simulink library "Ampere_Library"  (R2022b)
settings: Solver=FixedStepDiscrete  StartTime=0  StopTime=10.0  RelTol=1e-3  EnableMultiTasking=on
undefined symbols (not defined in the file or in its folder): A_INST_double, Dem_EventStatusType, ECU_AMBIENT_TEMPERATURE, SET_ECU_AMBIENT_TEMPERATURE, SlDemoSign, Std_ReturnType
libraries: simulink x13
(part 7 of 10)

== system Ampere_Library/User_Defined_Libraries/Discrete/A_1stOrder_Derivative_Filter ==
  note: A_DivisionByZero
  note: A_UnitDelayExternalIC
  note: Refer Mask Description of this Library block for detailed information.
  In : Inport
  Init_val : Inport  Port=2
  Tau : Inport  Port=3
  Te : Inport  Port=4
  Reset : Inport  Port=5
  Abs1 : Abs  RndMeth=Zero  SaturateOnIntegerOverflow=off
  ConstZero : Constant  Value=ConstZero  OutDataTypeStr=Inherit: Inherit via back propagation
  ConstZero1 : Constant  Value=ConstZero  OutDataTypeStr=Inherit: Inherit via back propagation
  Divide : Product  Inputs=*/  OutDataTypeStr=Inherit: Inherit via back propagation  RndMeth=Zero
  FixPtUnitDelay2 : UnitDelay  DisableCoverage=on  InitialCondition=false  SampleTime=-1  HasFrameUpgradeWarning=on
      settings: AttributesFormatString=Init = %<InitialCondition>
  FixPt_Unit_Delay1 : UnitDelay  DisableCoverage=on  InitialCondition=UDEIC_zero  SampleTime=-1  HasFrameUpgradeWarning=on
      settings: AttributesFormatString=Init = %<InitialCondition>
  Init : Switch  Criteria=u2 ~= 0  RndMeth=Zero  ZeroCross=off  SaturateOnIntegerOverflow=off
  LogicalOperator : Logic  Operator=OR  OutDataTypeStr=boolean
  MinMax1 : MinMax  Function=max  Inputs=2  InputSameDT=on  RndMeth=Zero
  Product : Product  InputSameDT=on  OutDataTypeStr=Inherit: Inherit via back propagation  RndMeth=Zero
  RelationalOperator : RelationalOperator  Operator=>  OutDataTypeStr=boolean  RndMeth=Zero
  Sum : Sum  InputSameDT=on  RndMeth=Zero
  Sum1 : Sum  Inputs=+-  InputSameDT=on  RndMeth=Zero
  Sum2 : Sum  InputSameDT=on  OutDataTypeStr=Inherit: Inherit via back propagation  RndMeth=Zero
  Switch : Switch  Criteria=u2 ~= 0  RndMeth=Zero  SaturateOnIntegerOverflow=off
  Switch2 : Switch  Criteria=u2 ~= 0  RndMeth=Zero  SaturateOnIntegerOverflow=off
  Switch3 : Switch  Criteria=u2 ~= 0  RndMeth=Zero  SaturateOnIntegerOverflow=off
  UnitDelay1 : UnitDelay  InitialCondition=true  SampleTime=-1  HasFrameUpgradeWarning=on
      settings: AttributesFormatString=Init = %<InitialCondition>
  false : Constant  Value=false
  tol : Constant  Value=tol  OutDataTypeStr=Inherit: Inherit via back propagation
  true : Constant  DisableCoverage=on  Value=true
  Out : Outport
  dOut_by_dt : Outport  Port=2
  wires:
  ConstZero1/1 -> Switch3/1
  Product/1 -> Sum2/1
  Init/1 -> Sum1/2, Sum2/2
  false/1 -> UnitDelay1/1
  UnitDelay1/1 -> LogicalOperator/1
  Sum2/1 -> Switch2/3
  Tau/1 -> Sum/1
  Sum/1 -> MinMax1/1
  Reset/1 -> LogicalOperator/2
  In/1 -> Sum1/1
  Switch3/1 -> dOut_by_dt/1
  Switch/1 -> Switch3/3, Product/1
  LogicalOperator/1 -> Switch2/2, Switch3/2
  Init_val/1 -> Init/3, [Init_val]
  FixPt_Unit_Delay1/1 -> Init/1
  FixPtUnitDelay2/1 -> Init/2
  true/1 -> FixPtUnitDelay2/1
  Switch2/1 -> FixPt_Unit_Delay1/1, Out/1
  Abs1/1 -> RelationalOperator/1
  MinMax1/1 -> Divide/2, Abs1/1
  ConstZero/1 -> Switch/3
  tol/1 -> RelationalOperator/2
  Divide/1 -> Switch/1
  RelationalOperator/1 -> Switch/2
  Sum1/1 -> Divide/1
  [Init_val] -> Switch2/1
  Te/1 -> Product/2, MinMax1/2, Sum/2

== system Ampere_Library/User_Defined_Libraries/Discrete/A_DiagnosticFilter ==
  note: Refer Mask Description of this Library block for detailed information.
  Reset : Inport  OutDataTypeStr=boolean
      settings: AttributesFormatString=DT = %<OutDataTypeStr>
  in : Inport  Port=2
  Diagnostic_Filter : Subsystem  TreatAsAtomicUnit=on
      settings: RTWSystemCode=Inline
  out : Outport
  DiagnosticStatus : Outport  Port=2
  wires:
  Reset/1 -> Diagnostic_Filter/Enable
  Diagnostic_Filter/2(DiagnosticStatus) -> DiagnosticStatus/1
  Diagnostic_Filter/1(out) -> out/1
  in/1 -> Diagnostic_Filter/1(in)

== system Ampere_Library/User_Defined_Libraries/Discrete/A_DiscreteInt_Ext_SAT ==
  note: Detect Increase
  note: Refer Mask Description of this Library block for detailed information.
  in : Inport
  reset : Inport  Port=2
  ic : Inport  Port=3
  Ts : Inport  Port=4
  sat_max : Inport  Port=5
  sat_min : Inport  Port=6
  Logical_Operator : Logic  OutDataTypeStr=boolean
  Logical_Operator1 : Logic  Operator=NOT  OutDataTypeStr=boolean
  MinMax : MinMax  Function=max  Inputs=2  InputSameDT=on  RndMeth=Zero
      settings: AttributesFormatString=SAT = %<SaturateOnIntegerOverflow>\n
  MinMax1 : MinMax  Inputs=2  InputSameDT=on  RndMeth=Zero
      settings: AttributesFormatString=SAT = %<SaturateOnIntegerOverflow>\n
  Product : Product  InputSameDT=on  OutDataTypeStr=Inherit: Inherit via back propagation  RndMeth=Zero
      settings: AttributesFormatString=SAT = %<SaturateOnIntegerOverflow>\n
  Sum1 : Sum  InputSameDT=on  RndMeth=Zero
      settings: AttributesFormatString=SAT = %<SaturateOnIntegerOverflow>
  Switch : Switch  Criteria=u2 ~= 0  RndMeth=Zero  SaturateOnIntegerOverflow=off
      settings: AttributesFormatString=SAT = %<SaturateOnIntegerOverflow>
  Unit_Delay : UnitDelay  InitialCondition=Input_IC  SampleTime=-1  HasFrameUpgradeWarning=on
      settings: AttributesFormatString=Init = %<InitialCondition>
  Unit_Delay1 : UnitDelay  InitialCondition=IniVal  SampleTime=-1  HasFrameUpgradeWarning=on
      settings: AttributesFormatString=Init = %<InitialCondition>\n
  Unit_Delay2 : UnitDelay  InitialCondition=false  SampleTime=-1  HasFrameUpgradeWarning=on
      settings: AttributesFormatString=Init = %<InitialCondition>\n
  out : Outport
  wires:
  sat_max/1 -> MinMax1/1
  Unit_Delay1/1 -> Sum1/2
  Product/1 -> Sum1/1
  Unit_Delay/1 -> Product/1
  Ts/1 -> Product/2
  in/1 -> Unit_Delay/1
  Logical_Operator1/1 -> Logical_Operator/2
  Unit_Delay2/1 -> Logical_Operator1/1
  reset/1 -> Logical_Operator/1, Unit_Delay2/1
  ic/1 -> Switch/1
  Sum1/1 -> Switch/3
  MinMax/1 -> MinMax1/2
  MinMax1/1 -> Unit_Delay1/1, out/1
  Switch/1 -> MinMax/2
  Logical_Operator/1 -> Switch/2
  sat_min/1 -> MinMax/1

== system Ampere_Library/User_Defined_Libraries/Discrete/A_DiscreteIntegrator ==
  note: Unused data depending
      | of mask configuration
  note: Refer Mask Description of this Library block for detailed information.
  note: tmp = in[k-1] * K * Ts
  note: y[k] = tmp + y[k-1]
  note: y[k]
  note: GotoTag updated through mask callback
  in : Inport
  reset : Inport  Port=2
  ic : Inport  Port=3
  DataTypeDuplicate : DataTypeDuplicate  NumInputPorts=4
  K : Constant  Value=K  OutDataTypeStr=Inherit: Inherit via back propagation
  Logical_Operator : Logic  OutDataTypeStr=boolean
  Logical_Operator1 : Logic  Operator=NOT  OutDataTypeStr=boolean
  Logical_Operator5 : Logic  Operator=OR  OutDataTypeStr=boolean
  MinMax : MinMax  Function=max  Inputs=2  InputSameDT=on  RndMeth=Zero
  MinMax1 : MinMax  Inputs=2  InputSameDT=on  RndMeth=Zero
  Product : Product  OutDataTypeStr=Inherit: Inherit via back propagation  RndMeth=Zero
  Product1 : Product  OutDataTypeStr=Inherit: Inherit via back propagation  RndMeth=Zero
  Sum1 : Sum  InputSameDT=on  RndMeth=Zero
  Switch : Switch  Criteria=u2 ~= 0  RndMeth=Zero  SaturateOnIntegerOverflow=off
  Terminator : Terminator
  Terminator1 : Terminator
  Ts : Constant  Value=Ts  OutDataTypeStr=Inherit: Inherit via back propagation
  Unit_Delay : UnitDelay  InitialCondition=IniVal  SampleTime=-1  HasFrameUpgradeWarning=on
      settings: AttributesFormatString=Init = %<InitialCondition>\n
  Unit_Delay1 : UnitDelay  InitialCondition=IniVal  SampleTime=-1  HasFrameUpgradeWarning=on
      settings: AttributesFormatString=Init = %<InitialCondition>\n
  Unit_Delay2 : UnitDelay  InitialCondition=false  SampleTime=-1  HasFrameUpgradeWarning=on
      settings: AttributesFormatString=Init = %<InitialCondition>\n
  sat_max : Constant  Value=sat_max  OutDataTypeStr=Inherit: Inherit via back propagation
  sat_min : Constant  Value=sat_min  OutDataTypeStr=Inherit: Inherit via back propagation
  out : Outport
  wires:
  Logical_Operator5/1 -> [ext_reset_or]
  Logical_Operator/1 -> [ext_reset_and]
  Switch/1 -> MinMax/1
  MinMax1/1 -> out/1, Unit_Delay1/1
  sat_max/1 -> MinMax1/1
  sat_min/1 -> MinMax/2
  MinMax/1 -> MinMax1/2
  Sum1/1 -> Switch/3
  ic/1 -> Switch/1
  reset/1 -> Logical_Operator5/2, Unit_Delay2/1, Logical_Operator/1
  Unit_Delay2/1 -> Logical_Operator5/1, Logical_Operator1/1
  Logical_Operator1/1 -> Logical_Operator/2
  in/1 -> DataTypeDuplicate/4, Unit_Delay/1
  Ts/1 -> DataTypeDuplicate/1, Product/2
  K/1 -> DataTypeDuplicate/3, Product1/2
  Unit_Delay/1 -> Product1/1
  Product1/1 -> DataTypeDuplicate/2, Product/1
  Product/1 -> Sum1/1
  Unit_Delay1/1 -> Sum1/2
  [ext_reset_or] -> Switch/2
  [ext_reset_and] -> Terminator/1
  [ext_reset_or] -> Terminator1/1

== system Ampere_Library/User_Defined_Libraries/Discrete/A_DownFreezing ==
  note: Refer Mask Description of this Library block for detailed information.
  in : Inport
  MinMax : MinMax  Inputs=2  InputSameDT=on  RndMeth=Zero
  Unit_Delay : UnitDelay  InitialCondition=init  SampleTime=-1  HasFrameUpgradeWarning=on
      settings: AttributesFormatString=Init = %<InitialCondition>
  out : Outport
  wires:
  in/1 -> MinMax/1
  MinMax/1 -> Unit_Delay/1, out/1
  Unit_Delay/1 -> MinMax/2

== system Ampere_Library/User_Defined_Libraries/Discrete/A_FILTER1ST ==
  note: Updated through Mask Callback
  note: Refer Mask Description of this Library block for detailed information.
  input : Inport
  filter_parameter : Inport  Port=2
  initial : Inport  Port=3  OutDataTypeStr=boolean
      settings: AttributesFormatString=DT = %<OutDataTypeStr>
  DataTypeConversion : DataTypeConversion  SaturateOnIntegerOverflow=off
  Product : Product  OutDataTypeStr=double  RndMeth=Zero
      settings: AttributesFormatString=DT = %<OutDataTypeStr>\n
  Saturation : Saturate  UpperLimit=Up  LowerLimit=Low  RndMeth=Zero
      settings: AttributesFormatString="Max =  %<UpperLimit>\\n Min = %<LowerLimit> \\n"
  Saturation1 : Saturate  UpperLimit=output_satmax  LowerLimit=output_satmin  RndMeth=Zero
      settings: AttributesFormatString="Max =  %<UpperLimit>\\n Min = %<LowerLimit> \\n"
  Sum : Sum  Inputs=+-  InputSameDT=on  RndMeth=Zero
  Sum1 : Sum  InputSameDT=on  RndMeth=Zero
  Switch1 : Switch  Criteria=u2 ~= 0  Threshold=0.5  RndMeth=Zero  SaturateOnIntegerOverflow=off
  UnitDelay : UnitDelay  InitialCondition=initial_value  SampleTime=-1  HasFrameUpgradeWarning=on
      settings: AttributesFormatString=Init = %<InitialCondition>\n
  output : Outport
  wires:
  DataTypeConversion/1 -> Switch1/1
  Saturation1/1 -> output/1
  Product/1 -> Sum1/1
  Sum/1 -> Product/1
  Saturation/1 -> Product/2
  UnitDelay/1 -> Sum1/2, Sum/2
  input/1 -> DataTypeConversion/1, Sum/1
  Switch1/1 -> Saturation1/1, UnitDelay/1
  initial/1 -> Switch1/2
  Sum1/1 -> Switch1/3
  filter_parameter/1 -> Saturation/1

== system Ampere_Library/User_Defined_Libraries/Discrete/A_FirstOrderClim ==
  note: Rounding_system
  note: Enable block created/deleted
      | through Mask Callback
  note: Properties updated through Mask Callback
  note: Refer Mask Description of this Library block for detailed information.
  note: A_ADivB
  note: Resolution_system
  In : Inport
  Init : Inport  Port=2
  T_by_Tau : Inport  Port=3
  enableport1 : EnablePort  StatesWhenEnabling=reset
      settings: AttributesFormatString=%<StatesWhenEnabling>
  Abs1 : Abs  RndMeth=Zero  SaturateOnIntegerOverflow=off
  Abs2 : Abs  RndMeth=Zero  SaturateOnIntegerOverflow=off
  DataTypeConversion3 : DataTypeConversion  SaturateOnIntegerOverflow=off
      settings: AttributesFormatString=SAT = %<SaturateOnIntegerOverflow>
  DataTypeDuplicate : DataTypeDuplicate
  Divide : Product  Inputs=*/  OutDataTypeStr=Inherit: Inherit via back propagation  RndMeth=Zero
  InitCondition : UnitDelay  InitialCondition=true  SampleTime=-1  HasFrameUpgradeWarning=on
      settings: AttributesFormatString=Init = %<InitialCondition>\n
  InitCondition1 : UnitDelay  InitialCondition=IniVal  SampleTime=-1  HasFrameUpgradeWarning=on
      settings: AttributesFormatString=Init = %<InitialCondition>\n
  Product : Product  RndMeth=Zero
  Product1 : Product  Inputs=**  RndMeth=Zero
      settings: AttributesFormatString=DT = %<OutDataTypeStr>
  Product2 : Product  OutDataTypeStr=uint32  RndMeth=Zero  SaturateOnIntegerOverflow=on
      settings: AttributesFormatString=SAT = %<SaturateOnIntegerOverflow>\n DT = %<OutDataTypeStr>\n
  Product3 : Product  Inputs=*/  RndMeth=Zero
  RF0 : Constant  Value=RF0  OutDataTypeStr=Inherit: Inherit via back propagation
  RF1 : Constant  Value=RF1  OutDataTypeStr=Inherit: Inherit via back propagation
  RF2 : Constant  Value=RF1  OutDataTypeStr=Inherit: Inherit via back propagation
  RF5 : Constant  Value=RF5  OutDataTypeStr=Inherit: Inherit via back propagation
  RelationalOperator : RelationalOperator  Operator=>  OutDataTypeStr=boolean  RndMeth=Zero
  RelationalOperator1 : RelationalOperator  OutDataTypeStr=boolean  RndMeth=Zero
  RelationalOperator4 : RelationalOperator  Operator=>  OutDataTypeStr=boolean  RndMeth=Zero
  Subtract10 : Sum  Inputs=-+  InputSameDT=on  RndMeth=Zero
  Subtract4 : Sum  Inputs=--  InputSameDT=on  RndMeth=Zero
  Subtract9 : Sum  InputSameDT=on  RndMeth=Zero
  Sum1 : Sum  InputSameDT=on  RndMeth=Zero
  Sum2 : Sum  InputSameDT=on  RndMeth=Zero
  Switch{,1..2,10} (4 alike) : Switch  Criteria=u2 ~= 0  RndMeth=Zero  SaturateOnIntegerOverflow=off
  contrl_value : Constant  Value=contrl_value  OutDataTypeStr=Inherit: Inherit via back propagation
  false : Constant  Value=false
  resolution : Constant  Value=resolution  OutDataTypeStr=Inherit: Inherit via back propagation
  tol : Constant  Value=tol  OutDataTypeStr=Inherit: Inherit via back propagation
  Out : Outport  OutputWhenDisabled=reset  InitialOutput=default_value
      settings: AttributesFormatString=|
      | %<OutputWhenDisabled>
      | Init = %<InitialOutput>
  wires:
  Switch10/1 -> Product1/1
  Product1/1 -> Out/1
  resolution/1 -> Product1/2, Product3/2, DataTypeDuplicate/2
  Product3/1 -> Abs2/1, RelationalOperator4/1  "Input"
  Switch2/1 -> Subtract9/2, Subtract4/2  "GreaterDcon"
  RelationalOperator1/1 -> Switch2/2
  RF5/1 -> RelationalOperator1/2
  Subtract10/1 -> RelationalOperator1/1  "Difference"
  [int_out] -> Subtract9/1
  [Check] -> Switch10/2
  Subtract4/1 -> Switch10/3
  [int_out] -> Subtract4/1
  RelationalOperator4/1 -> [Check]
  Product2/1 -> DataTypeConversion3/1
  RF0/1 -> RelationalOperator4/2, [Zero_out]
  RF2/1 -> [cons1], Product2/1
  Abs2/1 -> Subtract10/2, Product2/2
  Subtract9/1 -> Switch10/1
  [cons1] -> Switch2/1
  [Zero_out] -> Switch2/3
  DataTypeConversion3/1 -> Subtract10/1, [int_out]
  In/1 -> Product/1
  RelationalOperator/1 -> Switch1/2
  contrl_value/1 -> Switch1/3
  Abs1/1 -> RelationalOperator/1
  Sum2/1 -> Abs1/1, Switch1/1
  tol/1 -> RelationalOperator/2
  Sum1/1 -> Divide/1
  Switch1/1 -> Divide/2
  Divide/1 -> Switch/3
  Init/1 -> Switch/1
  Switch/1 -> Product3/1, DataTypeDuplicate/1, InitCondition1/1  "U"
  Product/1 -> Sum1/1
  false/1 -> InitCondition/1
  InitCondition/1 -> Switch/2
  T_by_Tau/1 -> Sum2/1, Product/2
  RF1/1 -> Sum2/2
  InitCondition1/1 -> Sum1/2  "U_z1"

== system Ampere_Library/User_Defined_Libraries/Discrete/A_InvalidValue ==
  note: Refer Mask Description of this Library block for detailed information.
  Constant : Constant  Value=InvalidValue
  Out : Outport
  wires:
  Constant/1 -> Out/1

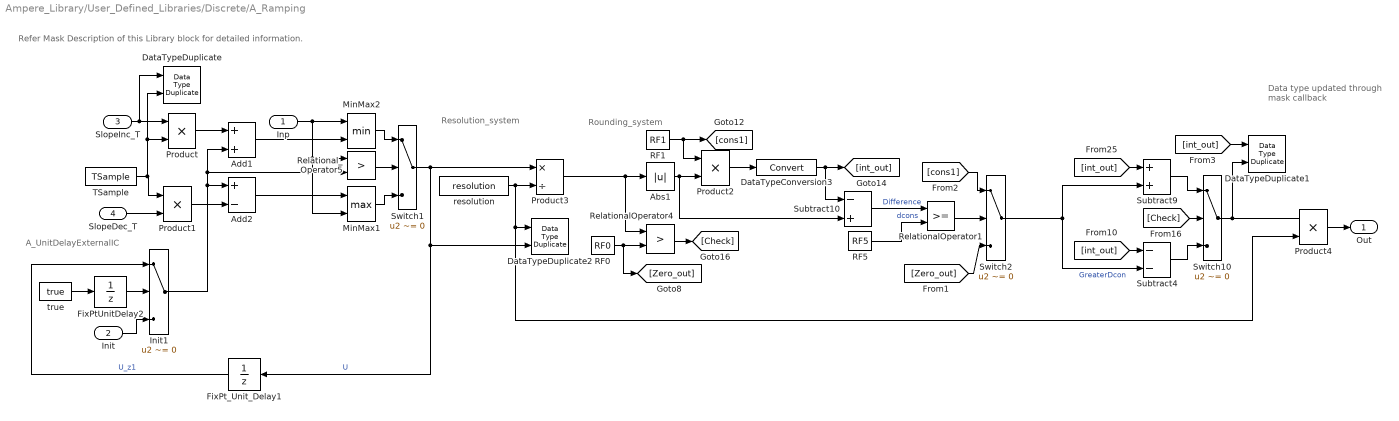
== system Ampere_Library/User_Defined_Libraries/Discrete/A_Ramping ==
  note: Rounding_system
  note: Refer Mask Description of this Library block for detailed information.
  note: A_UnitDelayExternalIC
  note: Resolution_system
  note: Data type updated
      | through mask callback
  Inp : Inport
  Init : Inport  Port=2
  SlopeInc_T : Inport  Port=3
  SlopeDec_T : Inport  Port=4
  Abs1 : Abs  RndMeth=Zero  SaturateOnIntegerOverflow=off
  Add1 : Sum  InputSameDT=on  RndMeth=Zero
  Add2 : Sum  Inputs=+-  InputSameDT=on  RndMeth=Zero
  DataTypeConversion3 : DataTypeConversion  SaturateOnIntegerOverflow=off
  DataTypeDuplicate : DataTypeDuplicate
  DataTypeDuplicate1 : DataTypeDuplicate
  DataTypeDuplicate2 : DataTypeDuplicate
  FixPtUnitDelay2 : UnitDelay  DisableCoverage=on  InitialCondition=false  SampleTime=-1  HasFrameUpgradeWarning=on
      settings: AttributesFormatString=Init = %<InitialCondition>
  FixPt_Unit_Delay1 : UnitDelay  DisableCoverage=on  InitialCondition=UDEIC_zero  SampleTime=-1  HasFrameUpgradeWarning=on
      settings: AttributesFormatString=Init = %<InitialCondition>
  Init1 : Switch  Criteria=u2 ~= 0  RndMeth=Zero  ZeroCross=off  SaturateOnIntegerOverflow=off
  MinMax1 : MinMax  Function=max  Inputs=2  InputSameDT=on  RndMeth=Zero
  MinMax2 : MinMax  Inputs=2  InputSameDT=on  RndMeth=Zero
  Product : Product  OutDataTypeStr=Inherit: Inherit via back propagation  RndMeth=Zero
  Product1 : Product  OutDataTypeStr=Inherit: Inherit via back propagation  RndMeth=Zero
  Product2 : Product  OutDataTypeStr=uint32  RndMeth=Zero  SaturateOnIntegerOverflow=on
      settings: AttributesFormatString=SAT = %<SaturateOnIntegerOverflow>\n DT = %<OutDataTypeStr>\n
  Product3 : Product  Inputs=*/  OutDataTypeStr=double  RndMeth=Zero
      settings: AttributesFormatString=DT = %<OutDataTypeStr>
  Product4 : Product  Inputs=**  OutDataTypeStr=Inherit: Inherit via back propagation  RndMeth=Zero
      settings: AttributesFormatString=SAT = %<SaturateOnIntegerOverflow>\nDT = %<OutDataTypeStr>\n
  RF0 : Constant  Value=RF0  OutDataTypeStr=Inherit: Inherit via back propagation
  RF1 : Constant  Value=RF1  OutDataTypeStr=Inherit: Inherit via back propagation
  RF5 : Constant  Value=RF5  OutDataTypeStr=Inherit: Inherit via back propagation
  RelationalOperator1 : RelationalOperator  OutDataTypeStr=boolean  RndMeth=Zero
  RelationalOperator4 : RelationalOperator  Operator=>  OutDataTypeStr=boolean  RndMeth=Zero
  Relational_Operator5 : RelationalOperator  Operator=>  OutDataTypeStr=boolean  ZeroCross=off  RndMeth=Zero
  Subtract10 : Sum  Inputs=-+  InputSameDT=on  RndMeth=Zero
  Subtract4 : Sum  Inputs=--  InputSameDT=on  RndMeth=Zero
  Subtract9 : Sum  InputSameDT=on  RndMeth=Zero
  Switch1 : Switch  Criteria=u2 ~= 0  RndMeth=Zero  SaturateOnIntegerOverflow=off
  Switch10 : Switch  Criteria=u2 ~= 0  RndMeth=Zero  SaturateOnIntegerOverflow=off
  Switch2 : Switch  Criteria=u2 ~= 0  RndMeth=Zero  SaturateOnIntegerOverflow=off
  TSample : Constant  Value=TSample  OutDataTypeStr=Inherit: Inherit via back propagation
  resolution : Constant  Value=resolution  OutDataTypeStr=Inherit: Inherit via back propagation
  true : Constant  DisableCoverage=on  Value=true
  Out : Outport
  wires:
  Switch10/1 -> DataTypeDuplicate1/2, Product4/1
  resolution/1 -> Product3/2, DataTypeDuplicate2/1, Product4/2
  RelationalOperator1/1 -> Switch2/2
  [int_out] -> DataTypeDuplicate1/1
  Switch2/1 -> Subtract9/2, Subtract4/2  "GreaterDcon"
  RF5/1 -> RelationalOperator1/2  "dcons"
  [int_out] -> Subtract9/1
  [Check] -> Switch10/2
  Subtract4/1 -> Switch10/3
  [int_out] -> Subtract4/1
  RelationalOperator4/1 -> [Check]
  DataTypeConversion3/1 -> Subtract10/1, [int_out]
  Product2/1 -> DataTypeConversion3/1
  RF0/1 -> RelationalOperator4/2, [Zero_out]
  Product3/1 -> Abs1/1, RelationalOperator4/1
  RF1/1 -> Product2/1, [cons1]
  Abs1/1 -> Subtract10/2, Product2/2
  Subtract10/1 -> RelationalOperator1/1  "Difference"
  Subtract9/1 -> Switch10/1
  [cons1] -> Switch2/1
  [Zero_out] -> Switch2/3
  MinMax2/1 -> Switch1/1
  SlopeInc_T/1 -> DataTypeDuplicate/1, Product/1
  Product4/1 -> Out/1
  Inp/1 -> MinMax1/2, Relational_Operator5/1, MinMax2/1
  Add2/1 -> MinMax1/1
  Init1/1 -> Add2/1, Relational_Operator5/2, Add1/2
  Product/1 -> Add1/1
  Product1/1 -> Add2/2
  TSample/1 -> Product1/1, Product/2, DataTypeDuplicate/2
  Switch1/1 -> Product3/1, DataTypeDuplicate2/2, FixPt_Unit_Delay1/1  "U"
  SlopeDec_T/1 -> Product1/2
  Relational_Operator5/1 -> Switch1/2
  Add1/1 -> MinMax2/2
  FixPtUnitDelay2/1 -> Init1/2
  MinMax1/1 -> Switch1/3
  FixPt_Unit_Delay1/1 -> Init1/1  "U_z1"
  Init/1 -> Init1/3
  true/1 -> FixPtUnitDelay2/1

== system Ampere_Library/User_Defined_Libraries/Discrete/A_Ramping_with_EnRst ==
  note: A_UnitDelayResettable
  note: Refer Mask Description of this Library block for detailed information.
  Inp : Inport
  Init : Inport  Port=2
  SlopeInc_T : Inport  Port=3
  SlopeDec_T : Inport  Port=4
  SampleTime : Inport  Port=5
  SlopeEna : Inport  Port=6  OutDataTypeStr=boolean
      settings: AttributesFormatString=DT = %<OutDataTypeStr>
  Reset : Inport  Port=7
  Add1 : Sum  InputSameDT=on  RndMeth=Zero
  Add2 : Sum  Inputs=+-  InputSameDT=on  RndMeth=Zero
  FixPtUnitDelay2 : UnitDelay  DisableCoverage=on  InitialCondition=true  SampleTime=-1  HasFrameUpgradeWarning=on
      settings: AttributesFormatString=Init = %<InitialCondition>\n
  FixPt_Unit_Delay1 : UnitDelay  DisableCoverage=on  InitialCondition=UDEIC_zero  SampleTime=-1  HasFrameUpgradeWarning=on
      settings: AttributesFormatString=Init = %<InitialCondition>\n
  LogicalOperator1 : Logic  Operator=OR  OutDataTypeStr=boolean
  MinMax1 : MinMax  Function=max  Inputs=2  InputSameDT=on  RndMeth=Zero
  MinMax2 : MinMax  Inputs=2  InputSameDT=on  RndMeth=Zero
  Product : Product  InputSameDT=on  OutDataTypeStr=Inherit: Inherit via back propagation  RndMeth=Zero
  Product1 : Product  InputSameDT=on  OutDataTypeStr=Inherit: Inherit via back propagation  RndMeth=Zero
  Relational_Operator5 : RelationalOperator  Operator=>  OutDataTypeStr=boolean  ZeroCross=off  RndMeth=Zero
  Switch : Switch  Criteria=u2 ~= 0  RndMeth=Zero  ZeroCross=off  SaturateOnIntegerOverflow=off
  Switch1 : Switch  Criteria=u2 ~= 0  RndMeth=Zero  SaturateOnIntegerOverflow=off
  Switch2 : Switch  Criteria=u2 ~= 0  RndMeth=Zero  SaturateOnIntegerOverflow=off
  false : Constant  DisableCoverage=on  Value=false
  out : Outport
  wires:
  SampleTime/1 -> Product1/1, Product/2
  Product1/1 -> Add2/2
  SlopeDec_T/1 -> Product1/2
  Product/1 -> Add1/2
  SlopeInc_T/1 -> Product/1
  MinMax2/1 -> Switch1/1
  Relational_Operator5/1 -> Switch1/2
  Add2/1 -> MinMax1/1
  Add1/1 -> MinMax2/1
  MinMax1/1 -> Switch1/3
  Switch/1 -> Add1/1, Add2/1, Relational_Operator5/2
  [Inp] -> MinMax2/2, Relational_Operator5/1
  SlopeEna/1 -> Switch2/2
  Switch1/1 -> Switch2/1
  Inp/1 -> MinMax1/2, Switch2/3, [Inp]
  LogicalOperator1/1 -> Switch/2
  Switch2/1 -> out/1, FixPt_Unit_Delay1/1
  Init/1 -> Switch/1
  false/1 -> FixPtUnitDelay2/1
  FixPtUnitDelay2/1 -> LogicalOperator1/1
  Reset/1 -> LogicalOperator1/2
  FixPt_Unit_Delay1/1 -> Switch/3

== system Ampere_Library/User_Defined_Libraries/Discrete/A_TappedDelay ==
  note: Unused data depending
      | of mask configuration
  note: Refer Mask Description of this Library block for detailed information.
  note: GotoTag updated through mask callback
  note: Signal Copy to avoid mismatch between the outport name and the From tag that is modified through mask callback
  In : Inport
  A_NoOfDelay : Constant  Value=A_NoOfDelay
  Add1 : Sum  InputSameDT=on  RndMeth=Zero  SaturateOnIntegerOverflow=on
      settings: AttributesFormatString=SAT = %<SaturateOnIntegerOverflow>
  Add2 : Sum  Inputs=-+  InputSameDT=on  RndMeth=Zero  SaturateOnIntegerOverflow=on
      settings: AttributesFormatString=SAT = %<SaturateOnIntegerOverflow>
  INIADD : Constant  Value=IniAdd
  Logical_Operator1 : Logic  Operator=OR  OutDataTypeStr=boolean
  Logical_Operator2 : Logic  Operator=NOT  OutDataTypeStr=boolean
  Mux : Mux  Inputs=[1 3]
      settings: AttributesFormatString=%<Inputs>
  Mux1 : Mux  Inputs=[1 4]
      settings: AttributesFormatString=%<Inputs>
  RelationalOperator : RelationalOperator  Operator===  OutDataTypeStr=boolean  RndMeth=Zero
  Selector : Selector  IndexOptions=Index vector (dialog)  Indices=Selector  OutputSizes=1
      settings: AttributesFormatString=%<IndexMode>\nIdx = %<Indices>
  Selector2 : Selector  IndexOptions=Index vector (dialog)  Indices=Append  OutputSizes=1
      settings: AttributesFormatString=%<IndexMode>\nIdx = %<Indices>
  Selector4 : Selector  IndexOptions=Index vector (dialog)  Indices=Order_Selec_Inv  OutputSizes=1
      settings: AttributesFormatString=%<IndexMode>\nIdx = %<Indices>
  Selector5 : Selector  IndexOptions=Index vector (dialog)  Indices=Order_Selec_Req  OutputSizes=1
      settings: AttributesFormatString=%<IndexMode>\nIdx = %<Indices>
  SignalConversion : SignalConversion  OverrideOpt=off
  Switch4 : Switch  Criteria=u2 ~= 0  RndMeth=Zero  SaturateOnIntegerOverflow=off
      settings: AttributesFormatString=SAT = %<SaturateOnIntegerOverflow>
  Terminator : Terminator
  Terminator1 : Terminator
  Unit_Delay : UnitDelay  InitialCondition=false  SampleTime=-1  HasFrameUpgradeWarning=on
      settings: AttributesFormatString=Init = %<InitialCondition>
  Unit_Delay1 : UnitDelay  InitialCondition=TapdIni  SampleTime=-1  HasFrameUpgradeWarning=on
      settings: AttributesFormatString=Init = %<InitialCondition>
  Unit_Delay3 : UnitDelay  InitialCondition=init_val  SampleTime=-1  HasFrameUpgradeWarning=on
      settings: AttributesFormatString=Init = %<InitialCondition>
  Unit_Delay4 : UnitDelay  InitialCondition=init_val  SampleTime=-1  HasFrameUpgradeWarning=on
      settings: AttributesFormatString=Init = %<InitialCondition>
  init_val : Constant  Value=init_val  OutDataTypeStr=Inherit: Inherit via back propagation
  Out : Outport
  wires:
  SignalConversion/1 -> Out/1
  [In] -> Mux1/1
  Logical_Operator1/1 -> Logical_Operator2/1, Unit_Delay/1
  Logical_Operator2/1 -> Switch4/2
  Selector/1 -> Mux/2
  [newest_order] -> SignalConversion/1
  Unit_Delay4/1 -> Mux/1
  RelationalOperator/1 -> Logical_Operator1/1
  In/1 -> Unit_Delay4/1, [In]
  Unit_Delay3/1 -> Selector/1
  A_NoOfDelay/1 -> RelationalOperator/2
  Add1/1 -> Unit_Delay1/1, Add2/2
  Add2/1 -> RelationalOperator/1
  Unit_Delay1/1 -> Add1/2
  Switch4/1 -> Mux1/2
  Selector2/1 -> Selector5/1, Selector4/1
  Mux/1 -> Switch4/3, Unit_Delay3/1
  [oldest_order] -> Terminator1/1
  [newest_order] -> Terminator/1
  Unit_Delay/1 -> Logical_Operator1/2
  Selector5/1 -> [newest_order]
  Selector4/1 -> [oldest_order]
  INIADD/1 -> Add2/1, Add1/1
  Mux1/1 -> Selector2/1
  init_val/1 -> Switch4/1

== system Ampere_Library/User_Defined_Libraries/Discrete/A_TimeDwnFrzSatOut ==
  note: DetectIncrease
  note: Refer Mask Description of this Library block for detailed information.
  Inp : Inport
  Add1 : Sum  Inputs=+-  InputSameDT=on  RndMeth=Zero
      settings: AttributesFormatString=SAT = %<SaturateOnIntegerOverflow>
  Add2 : Sum  InputSameDT=on  RndMeth=Zero
      settings: AttributesFormatString=SAT = %<SaturateOnIntegerOverflow>
  Demux : Demux  Outputs=2
  FreezedValue : Constant  Value=FreezedValue  OutDataTypeStr=Inherit: Inherit via back propagation
  InitialValue : Constant  Value=InitialValue  OutDataTypeStr=Inherit: Inherit via back propagation
  LogicalOperator : Logic  OutDataTypeStr=boolean
  LogicalOperator1 : Logic  OutDataTypeStr=boolean
  LogicalOperator2 : Logic  Operator=NOT  OutDataTypeStr=boolean
  LogicalOperator3 : Logic  Operator=NOT  OutDataTypeStr=boolean
  Mux : Mux  Inputs=2
  Mux1 : Mux  Inputs=2
  RelationalOperator1 : RelationalOperator  Operator=>  OutDataTypeStr=boolean  RndMeth=Zero
  RelationalOperator2 : RelationalOperator  Operator=>  OutDataTypeStr=boolean  RndMeth=Zero
  RelationalOperator4 : RelationalOperator  OutDataTypeStr=boolean  RndMeth=Zero
  ST : Constant  Value=ST  OutDataTypeStr=Inherit: Inherit via back propagation
  Switch{,1..4} (5 alike) : Switch  Criteria=u2 ~= 0  RndMeth=Zero  SaturateOnIntegerOverflow=off
      settings: AttributesFormatString=SAT = %<SaturateOnIntegerOverflow>
  UnitDelay : UnitDelay  InitialCondition=false  SampleTime=-1  HasFrameUpgradeWarning=on
      settings: AttributesFormatString=Init = %<InitialCondition>
  UnitDelay1 : UnitDelay  InitialCondition=false  SampleTime=-1  HasFrameUpgradeWarning=on
      settings: AttributesFormatString=Init = %<InitialCondition>
  UnitDelay{2..5} (4 alike) : UnitDelay  InitialCondition=IniVal  SampleTime=-1  HasFrameUpgradeWarning=on
      settings: AttributesFormatString=Init = %<InitialCondition>
  WaitInitTime : Constant  Value=WaitInitTime  OutDataTypeStr=Inherit: Inherit via back propagation
  true : Constant  Value=true
  Out : Outport
  wires:
  LogicalOperator2/1 -> LogicalOperator/2
  RelationalOperator4/1 -> UnitDelay1/1, Switch1/2, LogicalOperator/1
  Add2/1 -> UnitDelay2/1, Mux/2, Add1/1
  [Inp] -> Switch3/1, Switch4/1
  Switch3/1 -> Switch4/3
  Switch4/1 -> Switch1/1
  RelationalOperator1/1 -> LogicalOperator3/1, LogicalOperator1/2
  LogicalOperator3/1 -> Switch2/2
  LogicalOperator1/1 -> Switch3/2
  RelationalOperator2/1 -> LogicalOperator1/1
  Demux/2 -> UnitDelay4/1
  UnitDelay1/1 -> LogicalOperator2/1
  UnitDelay3/1 -> RelationalOperator2/1, Switch2/3, Switch1/3
  LogicalOperator/1 -> Switch4/2
  UnitDelay4/1 -> UnitDelay5/1, Add1/2
  Switch2/1 -> Switch3/3
  Inp/1 -> RelationalOperator1/1, [Inp], RelationalOperator2/2
  ST/1 -> Add2/1
  Mux1/1 -> Switch/1
  Switch1/1 -> Mux1/1
  Add1/1 -> RelationalOperator4/1
  Demux/1 -> Out/1, UnitDelay3/1
  Switch/1 -> Demux/1
  Mux/1 -> Switch/3
  InitialValue/1 -> Mux/1
  UnitDelay2/1 -> Add2/2
  FreezedValue/1 -> RelationalOperator1/2, Switch2/1
  WaitInitTime/1 -> RelationalOperator4/2
  UnitDelay/1 -> Switch/2
  true/1 -> UnitDelay/1
  UnitDelay5/1 -> Mux1/2

== system Ampere_Library/User_Defined_Libraries/Discrete/A_UnitDelayExternalIC ==
  note: Refer Mask Description of this Library block for detailed information.
  u : Inport
  IC : Inport  Port=2
  FixPtUnitDelay2 : UnitDelay  DisableCoverage=on  InitialCondition=false  SampleTime=-1  HasFrameUpgradeWarning=on
      settings: AttributesFormatString=Init = %<InitialCondition>
  FixPt_Unit_Delay1 : UnitDelay  DisableCoverage=on  InitialCondition=false  SampleTime=-1  HasFrameUpgradeWarning=on
      settings: AttributesFormatString=Init = %<InitialCondition>
  Init : Switch  Criteria=u2 ~= 0  RndMeth=Zero  ZeroCross=off  SaturateOnIntegerOverflow=off
      settings: AttributesFormatString=SAT = %<SaturateOnIntegerOverflow>
  true : Constant  DisableCoverage=on  Value=true
  y : Outport
  wires:
  u/1 -> FixPt_Unit_Delay1/1
  true/1 -> FixPtUnitDelay2/1
  FixPtUnitDelay2/1 -> Init/2
  Init/1 -> y/1
  FixPt_Unit_Delay1/1 -> Init/1
  IC/1 -> Init/3

== system Ampere_Library/User_Defined_Libraries/Discrete/A_UnitDelayResettable ==
  note: Refer Mask Description of this Library block for detailed information.
  u : Inport
  IC : Inport  Port=2
  Reset : Inport  Port=3
  FixPtUnitDelay2 : UnitDelay  DisableCoverage=on  InitialCondition=true  SampleTime=-1  HasFrameUpgradeWarning=on
      settings: AttributesFormatString=Init = %<InitialCondition>\n
  FixPt_Unit_Delay1 : UnitDelay  DisableCoverage=on  InitialCondition=UDEIC_zero  SampleTime=-1  HasFrameUpgradeWarning=on
      settings: AttributesFormatString=Init = %<InitialCondition>\n
  LogicalOperator1 : Logic  Operator=OR  OutDataTypeStr=boolean
  Switch : Switch  Criteria=u2 ~= 0  RndMeth=Zero  ZeroCross=off  SaturateOnIntegerOverflow=off
      settings: AttributesFormatString=SAT = %<SaturateOnIntegerOverflow>
  false : Constant  DisableCoverage=on  Value=false
  y : Outport
  wires:
  FixPt_Unit_Delay1/1 -> Switch/3
  Reset/1 -> LogicalOperator1/2
  FixPtUnitDelay2/1 -> LogicalOperator1/1
  LogicalOperator1/1 -> Switch/2
  false/1 -> FixPtUnitDelay2/1
  Switch/1 -> y/1
  IC/1 -> Switch/1
  u/1 -> FixPt_Unit_Delay1/1

== system Ampere_Library/User_Defined_Libraries/FlipFlop/A_SRFlipFlop_Mask_Cust ==
  note: Refer Mask Description of this Library block for detailed information.
  note: From tags and constant values are
      | reversed through mask callback
  Set : Inport
  ReSet : Inport  Port=2
  ConstantCb1 : Constant  Value=true
  ConstantCb2 : Constant  Value=false
  Switch1 : Switch  Criteria=u2 ~= 0  RndMeth=Zero  SaturateOnIntegerOverflow=off
  Switch3 : Switch  Criteria=u2 ~= 0  RndMeth=Zero  SaturateOnIntegerOverflow=off
  UnitDelay : UnitDelay  InitialCondition=IC  SampleTime=-1  HasFrameUpgradeWarning=on
      settings: AttributesFormatString=Init = %<InitialCondition>
  Out : Outport
  wires:
  [ReSet] -> Switch1/2
  [Set] -> Switch3/2
  ReSet/1 -> [ReSet]
  Set/1 -> [Set]
  UnitDelay/1 -> Switch1/3
  Switch3/1 -> UnitDelay/1, Out/1
  ConstantCb1/1 -> Switch3/1
  Switch1/1 -> Switch3/3
  ConstantCb2/1 -> Switch1/1

== system Ampere_Library/User_Defined_Libraries/FlipFlop/A_SRFlipFlop_indeter_F ==
  note: Refer Mask Description of this Library block for detailed information.
  set : Inport
  clear : Inport  Port=2
  AND : Logic  OutDataTypeStr=boolean
  NOT : Logic  Operator=NOT  OutDataTypeStr=boolean
  OR : Logic  Operator=OR  OutDataTypeStr=boolean
  UnitDelay : UnitDelay  InitialCondition=false  SampleTime=-1  HasFrameUpgradeWarning=on
      settings: AttributesFormatString=Init = %<InitialCondition>
  flag : Outport
  wires:
  OR/1 -> AND/2
  NOT/1 -> AND/1
  clear/1 -> NOT/1
  AND/1 -> UnitDelay/1, flag/1
  UnitDelay/1 -> OR/2
  set/1 -> OR/1

== system Ampere_Library/User_Defined_Libraries/Logic_and_Bit_Operations/A_CompareToConstant ==
  note: Refer Mask Description of this Library block for detailed information.
  u : Inport
  Compare : RelationalOperator  Operator===  OutDataTypeStr=boolean  ZeroCross=off  RndMeth=Zero
  Const : Constant  DisableCoverage=on  Value=Const  OutDataTypeStr=Inherit: Inherit via back propagation
  y : Outport
  wires:
  Compare/1 -> y/1
  Const/1 -> Compare/2
  u/1 -> Compare/1

== system Ampere_Library/User_Defined_Libraries/Logic_and_Bit_Operations/A_CompareToZero ==
  note: Refer Mask Description of this Library block for detailed information.
  u : Inport
  Compare : RelationalOperator  Operator===  OutDataTypeStr=boolean  ZeroCross=off  RndMeth=Zero
  cons_zero : Constant  DisableCoverage=on  Value=cons_zero  OutDataTypeStr=Inherit: Inherit via back propagation  PreserveConstantTs=on
  y : Outport
  wires:
  Compare/1 -> y/1
  u/1 -> Compare/1
  cons_zero/1 -> Compare/2

== system Ampere_Library/User_Defined_Libraries/Logic_and_Bit_Operations/A_DEDGE ==
  note: Refer Mask Description of this Library block for detailed information.
  flag : Inport
  LogicalOperator : Logic  OutDataTypeStr=boolean
  LogicalOperator1 : Logic  Operator=NOT  OutDataTypeStr=boolean
  UnitDelay : UnitDelay  InitialCondition=false  SampleTime=-1  HasFrameUpgradeWarning=on
      settings: AttributesFormatString=Init = %<InitialCondition>\n
  Fall : Outport
  wires:
  UnitDelay/1 -> LogicalOperator/2
  flag/1 -> LogicalOperator1/1, UnitDelay/1
  LogicalOperator/1 -> Fall/1
  LogicalOperator1/1 -> LogicalOperator/1

== system Ampere_Library/User_Defined_Libraries/Logic_and_Bit_Operations/A_DetectChange ==
  note: Refer Mask Description of this Library block for detailed information.
  U : Inport
  Float_CompInit : Subsystem  VariantControl=Float_CompInit
  Float_NoComp : Subsystem  VariantControl=Float_NoComp
  NonFloat_CompInit : Subsystem  VariantControl=NonFloat_CompInit
  NonFloat_NoComp : Subsystem  VariantControl=NonFloat_NoComp
  Y : Outport

== system Ampere_Library/User_Defined_Libraries/Logic_and_Bit_Operations/A_DetectIncDec ==
  note: Updated through
      | mask callback
  note: Refer Mask Description of this Library block for detailed information.
  note: Unused data depending
      | of the mask configuration
  U : Inport
  Delay_Input1 : UnitDelay  Description=Store in Global RAM  DisableCoverage=on  InitialCondition=vinit  SampleTime=-1  HasFrameUpgradeWarning=on
      settings: AttributesFormatString=Init = %<InitialCondition>\n
  Delay_Input2 : UnitDelay  Description=Store in Global RAM  DisableCoverage=on  InitialCondition=false  SampleTime=-1  HasFrameUpgradeWarning=on
      settings: AttributesFormatString=Init = %<InitialCondition>\n
  IncDec : RelationalOperator  Operator=<  OutDataTypeStr=boolean  ZeroCross=off  RndMeth=Zero
  Switch : Switch  Criteria=u2 ~= 0  RndMeth=Zero  SaturateOnIntegerOverflow=off
  Terminator : Terminator
  Terminator1 : Terminator
  false : Constant  Value=false
  true : Constant  Value=true
  Y : Outport
  wires:
  Delay_Input1/1 -> IncDec/2
  U/1 -> Delay_Input1/1, IncDec/1
  Delay_Input2/1 -> Switch/2
  false/1 -> [vchk_val]
  true/1 -> Delay_Input2/1
  [fromRelOpe] -> Switch/3
  IncDec/1 -> Switch/1, [fromRelOpe]
  [vchk_val] -> Terminator/1
  [fromRelOpe] -> Terminator1/1
  Switch/1 -> Y/1

== system Ampere_Library/User_Defined_Libraries/Logic_and_Bit_Operations/A_EdgeDetect_Ext_IC ==
  note: Unused data depending on the
      | mask configuration
  note: A_UnitDelayExternalIC
  note: Refer Mask Description of this Library block for detailed information.
  note: Updated through
      | mask callback
  In : Inport
  IC : Inport  Port=2
  Init : Switch  Criteria=u2 ~= 0  RndMeth=Zero  ZeroCross=off  SaturateOnIntegerOverflow=off
  InitOutVal : Constant  Value=false
  Logical_Operator : Logic  OutDataTypeStr=boolean
  Logical_Operator1 : Logic  Operator=NOT  OutDataTypeStr=boolean
  Logical_Operator2 : Logic  OutDataTypeStr=boolean
  Logical_Operator3 : Logic  Operator=NOT  OutDataTypeStr=boolean
  Logical_Operator4 : Logic  Operator=XOR  OutDataTypeStr=boolean
  SignalConversion : SignalConversion  OverrideOpt=off
  Switch : Switch  Criteria=u2 ~= 0  RndMeth=Zero  SaturateOnIntegerOverflow=off
  Terminator{,1..4} (5 alike) : Terminator
  UnitDelay2 : UnitDelay  DisableCoverage=on  InitialCondition=false  SampleTime=-1  HasFrameUpgradeWarning=on
      settings: AttributesFormatString=Init = %<InitialCondition>
  Unit_Delay1 : UnitDelay  DisableCoverage=on  InitialCondition=false  SampleTime=-1  HasFrameUpgradeWarning=on
      settings: AttributesFormatString=Init = %<InitialCondition>
  true1 : Constant  DisableCoverage=on  Value=true
  Out : Outport
  wires:
  [Either] -> Terminator2/1
  [FallingEdge] -> Terminator1/1
  [RisingEdge] -> Terminator/1
  Logical_Operator4/1 -> [Either]
  Logical_Operator2/1 -> [FallingEdge]
  Logical_Operator/1 -> [RisingEdge]
  [y] -> Logical_Operator4/2
  [y] -> Logical_Operator2/2
  [y] -> Logical_Operator1/1
  Init/1 -> [y]
  Logical_Operator3/1 -> Logical_Operator2/1
  Logical_Operator1/1 -> Logical_Operator/2
  [RisingEdge] -> Switch/1, SignalConversion/1
  InitOutVal/1 -> [vchk_val]
  [vchk_val] -> Switch/3
  [InitF] -> Switch/2
  Switch/1 -> Out/1
  [Check_Type] -> Terminator3/1
  [vchk_val] -> Terminator4/1
  IC/1 -> Init/3
  Unit_Delay1/1 -> Init/1
  UnitDelay2/1 -> Init/2, [InitF]
  true1/1 -> UnitDelay2/1
  In/1 -> Logical_Operator/1, Logical_Operator3/1, Logical_Operator4/1, Unit_Delay1/1
  SignalConversion/1 -> [Check_Type]

== system Ampere_Library/User_Defined_Libraries/Logic_and_Bit_Operations/A_Either_EdgeDetect ==
  note: Refer Mask Description of this Library block for detailed information.
  flag : Inport
  LogicalOperator : Logic  Operator=XOR  AllPortsSameDT=off  OutDataTypeStr=boolean
  UnitDelay : UnitDelay  InitialCondition=false  SampleTime=-1  HasFrameUpgradeWarning=on
      settings: AttributesFormatString=Init = %<InitialCondition>\n
  Either : Outport
  wires:
  UnitDelay/1 -> LogicalOperator/2
  flag/1 -> LogicalOperator/1, UnitDelay/1
  LogicalOperator/1 -> Either/1

== system Ampere_Library/User_Defined_Libraries/Logic_and_Bit_Operations/A_UEDGE ==
  note: Refer Mask Description of this Library block for detailed information.
  flag : Inport
  LogicalOperator : Logic  OutDataTypeStr=boolean
  LogicalOperator1 : Logic  Operator=NOT  OutDataTypeStr=boolean
  UnitDelay : UnitDelay  InitialCondition=false  SampleTime=-1  HasFrameUpgradeWarning=on
      settings: AttributesFormatString=Init = %<InitialCondition>\n
  Rise : Outport
  wires:
  UnitDelay/1 -> LogicalOperator1/1
  flag/1 -> LogicalOperator/1, UnitDelay/1
  LogicalOperator/1 -> Rise/1
  LogicalOperator1/1 -> LogicalOperator/2

== system Ampere_Library/User_Defined_Libraries/Lookup_Tables/A_Carto1D ==
  note: Refer Mask Description of this Library block for detailed information.
  note: Use native "One_D_Lookup_Table" block available in MBD_Base_Blocks/Simulink/Lookup_Tables
  Var : Inport
  data_1D_Lookup_Table : Lookup_n-D  NumberOfTableDimensions=1  BreakpointsForDimension1=x  Table=z  ExtrapMethod=Clip  UseLastTableValue=on  OutDataTypeStr=Inherit: Inherit from 'Table data'  RndMeth=Zero
      settings: AttributesFormatString=|
      | Table = %<Table>
      | X = %<BreakpointsForDimension1>
      | SAT = %<SaturateOnIntegerOverflow>
  Result : Outport
  wires:
  Var/1 -> data_1D_Lookup_Table/1
  data_1D_Lookup_Table/1 -> Result/1

== system Ampere_Library/User_Defined_Libraries/Lookup_Tables/A_Carto2D ==
  note: Refer Mask Description of this Library block for detailed information.
  note: Use native "Two_D_Lookup_Table" block available in MBD_Base_Blocks/Simulink/Lookup_Tables
  Var_x : Inport
  Var_y : Inport  Port=2
  LookupTable2D : Lookup_n-D  BreakpointsForDimension1=map_x  BreakpointsForDimension2=map_y  Table=carto  ExtrapMethod=Clip  UseLastTableValue=on  OutDataTypeStr=Inherit: Inherit from 'Table data'  RndMeth=Zero
      settings: InputPortMap=u0,u1
      settings: AttributesFormatString=|
      | Table = %<Table>
      | X = %<BreakpointsForDimension1>
      | Y = %<BreakpointsForDimension2>
      | Input same DT = %<InputSameDT>
      | SAT = %<SaturateOnIntegerOverflow>
  Result : Outport
  wires:
  Var_x/1 -> LookupTable2D/1
  Var_y/1 -> LookupTable2D/2
  LookupTable2D/1 -> Result/1

== system Ampere_Library/User_Defined_Libraries/Lookup_Tables/A_Cosine ==
  note: Refer Mask Description of this Library block for detailed information.
  u : Inport
  Amp25 : Sum  Inputs=+-  InputSameDT=on  RndMeth=Zero  SaturateOnIntegerOverflow=on  LockScale=on
      settings: AttributesFormatString=SAT = %<SaturateOnIntegerOverflow>\n
  Amp75 : Sum  Inputs=+-  InputSameDT=on  RndMeth=Zero  SaturateOnIntegerOverflow=on  LockScale=on
      settings: AttributesFormatString=SAT = %<SaturateOnIntegerOverflow>\n
  CONS_M1 : Constant  Value=Cons_M1  OutDataTypeStr=Inherit: Inherit via back propagation
  CONS_P25 : Constant  Value=Cons_P25  OutDataTypeStr=fixdt(0, OutputWordLength, OutputWordLength)
      settings: AttributesFormatString=DT = %<OutDataTypeStr>\n
  CONS_P5 : Constant  Value=Cons_P5  OutDataTypeStr=fixdt(0, OutputWordLength, OutputWordLength)
      settings: AttributesFormatString=DT = %<OutDataTypeStr>\n
  CONS_P75 : Constant  Value=Cons_P75  OutDataTypeStr=fixdt(0, OutputWordLength, OutputWordLength)
      settings: AttributesFormatString=DT = %<OutDataTypeStr>\n
  DataTypeConversion : DataTypeConversion  OutDataTypeStr=fixdt(0, OutputWordLength, OutputWordLength)
      settings: AttributesFormatString=SAT = %<SaturateOnIntegerOverflow>\n DT = %<OutDataTypeStr>\n
  DataTypeDuplicate : DataTypeDuplicate
  DataTypeDuplicate1 : DataTypeDuplicate
  DataTypeDuplicate2 : DataTypeDuplicate
  GTEp75 : RelationalOperator  OutDataTypeStr=boolean  ZeroCross=off  RndMeth=Zero
  LTEp25 : RelationalOperator  Operator=<=  OutDataTypeStr=boolean  ZeroCross=off  RndMeth=Zero
  LTEp50 : RelationalOperator  Operator=<=  OutDataTypeStr=boolean  ZeroCross=off  RndMeth=Zero
  LookupTable1_D : Lookup_n-D  NumberOfTableDimensions=1  BreakpointsForDimension1=k  BeginIndexSearchUsingPreviousIndexResult=on  Table=b  ExtrapMethod=Clip  UseLastTableValue=on  OutDataTypeStr=fixdt(1, OutputWordLength, OutputFracLength)  RndMeth=Zero  SaturateOnIntegerOverflow=on  FractionDataTypeStr=double
      settings: AttributesFormatString=Table = %<Table>\n X = %<BreakpointsForDimension1>\n
  Product2 : Product  OutDataTypeStr=Inherit: Inherit via back propagation  RndMeth=Zero  SaturateOnIntegerOverflow=on
      settings: AttributesFormatString=SAT = %<SaturateOnIntegerOverflow>\n
  QuadHandle1a : Switch  Criteria=u2 ~= 0  RndMeth=Zero  ZeroCross=off
      settings: AttributesFormatString=SAT = %<SaturateOnIntegerOverflow>
  QuadHandle1b : Switch  Criteria=u2 ~= 0  RndMeth=Zero  ZeroCross=off
      settings: AttributesFormatString=SAT = %<SaturateOnIntegerOverflow>
  QuadHandle2 : Switch  Criteria=u2 ~= 0  RndMeth=Zero  ZeroCross=off
      settings: AttributesFormatString=SAT = %<SaturateOnIntegerOverflow>
  SignCorrected : Switch  Criteria=u2 ~= 0  RndMeth=Zero  ZeroCross=off
      settings: AttributesFormatString=SAT = %<SaturateOnIntegerOverflow>
  firstor4thQuad : Logic  Operator=OR  OutDataTypeStr=boolean
  p25mA : Sum  Inputs=+-  InputSameDT=on  RndMeth=Zero  SaturateOnIntegerOverflow=on  LockScale=on
      settings: AttributesFormatString=SAT = %<SaturateOnIntegerOverflow>\n
  p75mA : Sum  Inputs=+-  InputSameDT=on  RndMeth=Zero  SaturateOnIntegerOverflow=on  LockScale=on
      settings: AttributesFormatString=SAT = %<SaturateOnIntegerOverflow>\n
  y : Outport
  wires:
  u/1 -> DataTypeConversion/1
  DataTypeConversion/1 -> LTEp25/1, p25mA/2, DataTypeDuplicate/2, p75mA/2, GTEp75/1, Amp75/1, LTEp50/1, Amp25/1
  LTEp25/1 -> QuadHandle1a/2, [firstquad]
  p25mA/1 -> DataTypeDuplicate2/2, QuadHandle1a/1
  Amp25/1 -> QuadHandle1a/3
  CONS_P25/1 -> [Point25]
  [Point25] -> LTEp25/2
  [Point25] -> Amp25/2
  [Point25] -> DataTypeDuplicate2/1, p25mA/1
  GTEp75/1 -> QuadHandle1b/2, [fourthquad]
  Amp75/1 -> QuadHandle1b/1
  CONS_P75/1 -> [Point75]
  [Point75] -> GTEp75/2, p75mA/1
  [Point75] -> Amp75/2
  p75mA/1 -> DataTypeDuplicate/1, QuadHandle1b/3
  CONS_P5/1 -> LTEp50/2
  LTEp50/1 -> QuadHandle2/2
  QuadHandle1a/1 -> QuadHandle2/1
  firstor4thQuad/1 -> SignCorrected/2
  [firstquad] -> firstor4thQuad/1
  [fourthquad] -> firstor4thQuad/2
  LookupTable1_D/1 -> Product2/1, DataTypeDuplicate1/1, SignCorrected/1
  Product2/1 -> SignCorrected/3
  SignCorrected/1 -> y/1
  CONS_M1/1 -> Product2/2, DataTypeDuplicate1/2
  QuadHandle2/1 -> LookupTable1_D/1
  QuadHandle1b/1 -> QuadHandle2/3
